simulink model "Lab7simu"  (R2017b)
settings: Solver=VariableStepAuto  StartTime=0.0  StopTime=50  RelTol=1e-3
values from neighbouring files (symbols this model uses):
  kd = eval(S.kd)    [Lab7.m]
  kd2 = eval(S.kd2)    [Lab7.m]
  ki = eval(S.ki)    [Lab7.m]
  kp = eval(S.kp)    [Lab7.m]
  tm = ts/40    (= 0.75)    [Lab7.m]
libraries: simulink x2
settings Model: Creator=Cx001la  LastModifiedBy=Cx001la

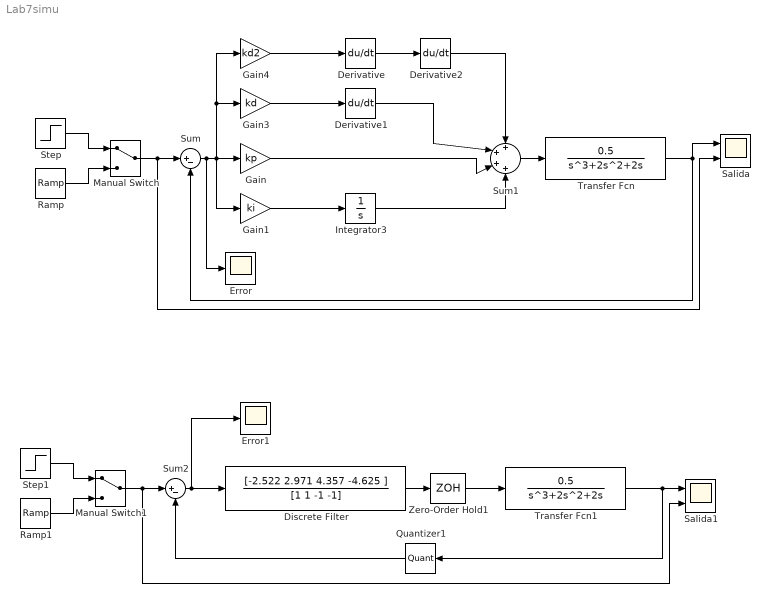
== system Lab7simu ==
  Derivative : Derivative
  Derivative1 : Derivative
  Derivative2 : Derivative
  Discrete Filter : DiscreteFilter  Numerator=[-2.522 2.971 4.357 -4.625 ]  Denominator=[1 1 -1 -1]  SampleTime=tm
  Error : Scope
  Error1 : Scope
  Gain : Gain  Gain=kp
  Gain1 : Gain  Gain=ki
  Gain3 : Gain  Gain=kd
  Gain4 : Gain  Gain=kd2
  Integrator3 : Integrator
  Manual Switch : ManualSwitch
  Manual Switch1 : ManualSwitch
  Quantizer1 : Quantizer  QuantizationInterval=1/1024
  Ramp : simulink/Sources/Ramp  slope=1  start=0  X0=0
  Ramp1 : simulink/Sources/Ramp  slope=1  start=0  X0=0
  Salida : Scope  NumInputPorts=2
  Salida1 : Scope  NumInputPorts=2
  Step : Step  Time=0  SampleTime=0
  Step1 : Step  Time=0  SampleTime=0
  Sum : Sum  Inputs=|+-
  Sum1 : Sum  Inputs=++++
  Sum2 : Sum  Inputs=|+-
  Transfer Fcn : TransferFcn  Numerator=[0.5]  Denominator=[1 2 2 0]
  Transfer Fcn1 : TransferFcn  Numerator=[0.5]  Denominator=[1 2 2 0]
  Zero-Order Hold1 : ZeroOrderHold  SampleTime=tm
  wires:
  Sum/1 -> Error/1, Gain1/1, Gain4/1, Gain3/1, Gain/1
  Gain1/1 -> Integrator3/1
  Gain3/1 -> Derivative1/1
  Gain/1 -> Sum1/3
  Derivative2/1 -> Sum1/1
  Integrator3/1 -> Sum1/4
  Sum1/1 -> Transfer Fcn/1
  Transfer Fcn/1 -> Sum/2, Salida/1
  Step/1 -> Manual Switch/1
  Manual Switch/1 -> Salida/2, Sum/1
  Ramp/1 -> Manual Switch/2
  Step1/1 -> Manual Switch1/1
  Sum2/1 -> Error1/1, Discrete Filter/1
  Manual Switch1/1 -> Salida1/2, Sum2/1
  Ramp1/1 -> Manual Switch1/2
  Discrete Filter/1 -> Zero-Order Hold1/1
  Transfer Fcn1/1 -> Quantizer1/1, Salida1/1
  Derivative/1 -> Derivative2/1
  Gain4/1 -> Derivative/1
  Derivative1/1 -> Sum1/2
  Zero-Order Hold1/1 -> Transfer Fcn1/1
  Quantizer1/1 -> Sum2/2
